simulink model "MBSE_system"  (R2022b)
settings: Solver=FixedStepDiscrete  StartTime=0.0  StopTime=10.0  RelTol=1e-3
settings Model: Creator=curro  LastModifiedBy=curro

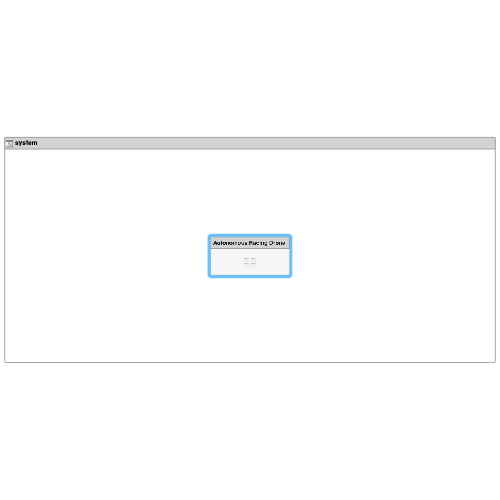
[thumbnail: Simulink's stored preview of the top-level diagram]
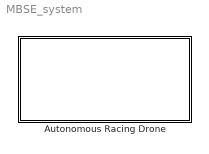
== system MBSE_system ==
  Autonomous Racing Drone : Subsystem
      settings: PortSchema="{\"entries\":[{\"content\":{\"headerSize\":26,\"margin\":15,\"minimumSpacing\":25,\"sides\":[{\"content\":{\"connectorIds\":[]},\"type\":\"ConnectorPlacement.EquallySpacedRectSide\",\"uuid\":\"710bb091-7129-4ee7-a780-76ad6f160d90\"},{\"content\":{\"connectorIds\":[],\"side\":\"RIGHT\"},\"type\":\"ConnectorPlacement.EquallySpacedRectSide\",\"uuid\":\"a14cb0ec-5ed5-4fd8-9e8a-b2c1d3079cde\"},{\"content\":{\"connectorIds\":[],\"side\":\"TOP\"},\"type\":\"ConnectorPlacement.EquallySpacedRectSide\",\"uuid\":\"b6825dff-2cae-452e-9344-6fbe12db9612\"}]},\"type\":\"ConnectorPlacement.EquallySpacedConnector\",\"uuid\":\"6fabdfc3-bcd5-4976-8a44-a7a5a39dd61e\"}],\"packageUris\":[\"http://schema.mathworks.com/mf0/Connector/R2020b\"],\"version\":\"1.0\"}"

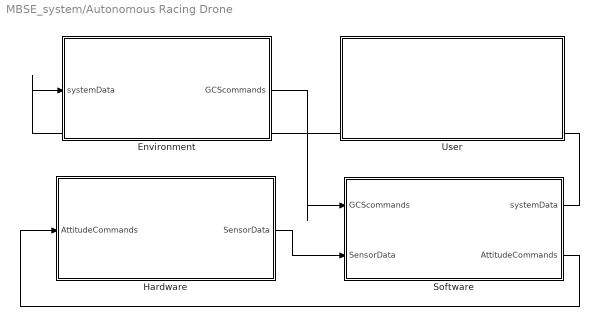
== system MBSE_system/Autonomous Racing Drone ==
  Environment : Subsystem
      settings: PortSchema="{\"entries\":[{\"content\":{\"headerSize\":26,\"margin\":15,\"minimumSpacing\":25,\"sides\":[{\"content\":{\"connectorIds\":[\"In1\"]},\"type\":\"ConnectorPlacement.EquallySpacedRectSide\",\"uuid\":\"710bb091-7129-4ee7-a780-76ad6f160d90\"},{\"content\":{\"connectorIds\":[\"Out1\"],\"side\":\"RIGHT\"},\"type\":\"ConnectorPlacement.EquallySpacedRectSide\",\"uuid\":\"a14cb0ec-5ed5-4fd8-9e8a-b2c1d3079cde\"},{\"content\":{\"connectorIds\":[],\"side\":\"TOP\"},\"type\":\"ConnectorPlacement.EquallySpacedRectSide\",\"uuid\":\"b6825dff-2cae-452e-9344-6fbe12db9612\"}]},\"type\":\"ConnectorPlacement.EquallySpacedConnector\",\"uuid\":\"6fabdfc3-bcd5-4976-8a44-a7a5a39dd61e\"}],\"packageUris\":[\"http://schema.mathworks.com/mf0/Connector/R2020b\"],\"version\":\"1.0\"}"
  Hardware : Subsystem
      settings: PortSchema="{\"entries\":[{\"content\":{\"headerSize\":26,\"margin\":15,\"minimumSpacing\":25,\"sides\":[{\"content\":{\"connectorIds\":[\"In1\"]},\"type\":\"ConnectorPlacement.EquallySpacedRectSide\",\"uuid\":\"710bb091-7129-4ee7-a780-76ad6f160d90\"},{\"content\":{\"connectorIds\":[\"Out1\"],\"side\":\"RIGHT\"},\"type\":\"ConnectorPlacement.EquallySpacedRectSide\",\"uuid\":\"a14cb0ec-5ed5-4fd8-9e8a-b2c1d3079cde\"},{\"content\":{\"connectorIds\":[],\"side\":\"TOP\"},\"type\":\"ConnectorPlacement.EquallySpacedRectSide\",\"uuid\":\"b6825dff-2cae-452e-9344-6fbe12db9612\"}]},\"type\":\"ConnectorPlacement.EquallySpacedConnector\",\"uuid\":\"6fabdfc3-bcd5-4976-8a44-a7a5a39dd61e\"}],\"packageUris\":[\"http://schema.mathworks.com/mf0/Connector/R2020b\"],\"version\":\"1.0\"}"
  Software : Subsystem
      settings: PortSchema="{\"entries\":[{\"content\":{\"headerSize\":26,\"margin\":15,\"minimumSpacing\":25,\"sides\":[{\"content\":{\"connectorIds\":[\"In2\",\"In1\"]},\"type\":\"ConnectorPlacement.EquallySpacedRectSide\",\"uuid\":\"710bb091-7129-4ee7-a780-76ad6f160d90\"},{\"content\":{\"connectorIds\":[\"Out1\",\"Out2\"],\"side\":\"RIGHT\"},\"type\":\"ConnectorPlacement.EquallySpacedRectSide\",\"uuid\":\"a14cb0ec-5ed5-4fd8-9e8a-b2c1d3079cde\"},{\"content\":{\"connectorIds\":[],\"side\":\"TOP\"},\"type\":\"ConnectorPlacement.EquallySpacedRectSide\",\"uuid\":\"b6825dff-2cae-452e-9344-6fbe12db9612\"}]},\"type\":\"ConnectorPlacement.EquallySpacedConnector\",\"uuid\":\"6fabdfc3-bcd5-4976-8a44-a7a5a39dd61e\"}],\"packageUris\":[\"http://schema.mathworks.com/mf0/Connector/R2020b\"],\"version\":\"1.0\"}"
  User : Subsystem
      settings: PortSchema="{\"entries\":[{\"content\":{\"headerSize\":26,\"margin\":15,\"minimumSpacing\":25,\"sides\":[{\"content\":{\"connectorIds\":[]},\"type\":\"ConnectorPlacement.EquallySpacedRectSide\",\"uuid\":\"710bb091-7129-4ee7-a780-76ad6f160d90\"},{\"content\":{\"connectorIds\":[],\"side\":\"RIGHT\"},\"type\":\"ConnectorPlacement.EquallySpacedRectSide\",\"uuid\":\"a14cb0ec-5ed5-4fd8-9e8a-b2c1d3079cde\"},{\"content\":{\"connectorIds\":[],\"side\":\"TOP\"},\"type\":\"ConnectorPlacement.EquallySpacedRectSide\",\"uuid\":\"b6825dff-2cae-452e-9344-6fbe12db9612\"}]},\"type\":\"ConnectorPlacement.EquallySpacedConnector\",\"uuid\":\"6fabdfc3-bcd5-4976-8a44-a7a5a39dd61e\"}],\"packageUris\":[\"http://schema.mathworks.com/mf0/Connector/R2020b\"],\"version\":\"1.0\"}"
  wires:
  Hardware/1(SensorData) -> Software/1(SensorData)
  Software/2(AttitudeCommands) -> Hardware/1(AttitudeCommands)
  Environment/1(GCScommands) -> Software/2(GCScommands)
  Software/1(systemData) -> Environment/1(systemData)

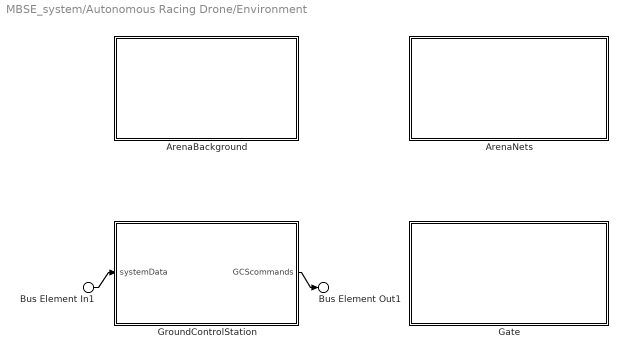
== system MBSE_system/Autonomous Racing Drone/Environment ==
  Bus Element In1 : Inport  PortName=systemData
  ArenaBackground : Subsystem
      settings: PortSchema="{\"entries\":[{\"content\":{\"headerSize\":26,\"margin\":15,\"minimumSpacing\":25,\"sides\":[{\"content\":{\"connectorIds\":[]},\"type\":\"ConnectorPlacement.EquallySpacedRectSide\",\"uuid\":\"710bb091-7129-4ee7-a780-76ad6f160d90\"},{\"content\":{\"connectorIds\":[],\"side\":\"RIGHT\"},\"type\":\"ConnectorPlacement.EquallySpacedRectSide\",\"uuid\":\"a14cb0ec-5ed5-4fd8-9e8a-b2c1d3079cde\"},{\"content\":{\"connectorIds\":[],\"side\":\"TOP\"},\"type\":\"ConnectorPlacement.EquallySpacedRectSide\",\"uuid\":\"b6825dff-2cae-452e-9344-6fbe12db9612\"}]},\"type\":\"ConnectorPlacement.EquallySpacedConnector\",\"uuid\":\"6fabdfc3-bcd5-4976-8a44-a7a5a39dd61e\"}],\"packageUris\":[\"http://schema.mathworks.com/mf0/Connector/R2020b\"],\"version\":\"1.0\"}"
  ArenaNets : Subsystem
      settings: PortSchema="{\"entries\":[{\"content\":{\"headerSize\":26,\"margin\":15,\"minimumSpacing\":25,\"sides\":[{\"content\":{\"connectorIds\":[]},\"type\":\"ConnectorPlacement.EquallySpacedRectSide\",\"uuid\":\"710bb091-7129-4ee7-a780-76ad6f160d90\"},{\"content\":{\"connectorIds\":[],\"side\":\"RIGHT\"},\"type\":\"ConnectorPlacement.EquallySpacedRectSide\",\"uuid\":\"a14cb0ec-5ed5-4fd8-9e8a-b2c1d3079cde\"},{\"content\":{\"connectorIds\":[],\"side\":\"TOP\"},\"type\":\"ConnectorPlacement.EquallySpacedRectSide\",\"uuid\":\"b6825dff-2cae-452e-9344-6fbe12db9612\"}]},\"type\":\"ConnectorPlacement.EquallySpacedConnector\",\"uuid\":\"6fabdfc3-bcd5-4976-8a44-a7a5a39dd61e\"}],\"packageUris\":[\"http://schema.mathworks.com/mf0/Connector/R2020b\"],\"version\":\"1.0\"}"
  Gate : Subsystem
      settings: PortSchema="{\"entries\":[{\"content\":{\"headerSize\":26,\"margin\":15,\"minimumSpacing\":25,\"sides\":[{\"content\":{\"connectorIds\":[]},\"type\":\"ConnectorPlacement.EquallySpacedRectSide\",\"uuid\":\"710bb091-7129-4ee7-a780-76ad6f160d90\"},{\"content\":{\"connectorIds\":[],\"side\":\"RIGHT\"},\"type\":\"ConnectorPlacement.EquallySpacedRectSide\",\"uuid\":\"a14cb0ec-5ed5-4fd8-9e8a-b2c1d3079cde\"},{\"content\":{\"connectorIds\":[],\"side\":\"TOP\"},\"type\":\"ConnectorPlacement.EquallySpacedRectSide\",\"uuid\":\"b6825dff-2cae-452e-9344-6fbe12db9612\"}]},\"type\":\"ConnectorPlacement.EquallySpacedConnector\",\"uuid\":\"6fabdfc3-bcd5-4976-8a44-a7a5a39dd61e\"}],\"packageUris\":[\"http://schema.mathworks.com/mf0/Connector/R2020b\"],\"version\":\"1.0\"}"
  GroundControlStation : Subsystem
      settings: PortSchema="{\"entries\":[{\"content\":{\"headerSize\":26,\"margin\":15,\"minimumSpacing\":25,\"sides\":[{\"content\":{\"connectorIds\":[\"In1\"]},\"type\":\"ConnectorPlacement.EquallySpacedRectSide\",\"uuid\":\"710bb091-7129-4ee7-a780-76ad6f160d90\"},{\"content\":{\"connectorIds\":[\"Out1\"],\"side\":\"RIGHT\"},\"type\":\"ConnectorPlacement.EquallySpacedRectSide\",\"uuid\":\"a14cb0ec-5ed5-4fd8-9e8a-b2c1d3079cde\"},{\"content\":{\"connectorIds\":[],\"side\":\"TOP\"},\"type\":\"ConnectorPlacement.EquallySpacedRectSide\",\"uuid\":\"b6825dff-2cae-452e-9344-6fbe12db9612\"}]},\"type\":\"ConnectorPlacement.EquallySpacedConnector\",\"uuid\":\"6fabdfc3-bcd5-4976-8a44-a7a5a39dd61e\"}],\"packageUris\":[\"http://schema.mathworks.com/mf0/Connector/R2020b\"],\"version\":\"1.0\"}"
  Bus Element Out1 : Outport  PortName=GCScommands
  wires:
  GroundControlStation/1(GCScommands) -> Bus Element Out1/1
  Bus Element In1/1 -> GroundControlStation/1(systemData)

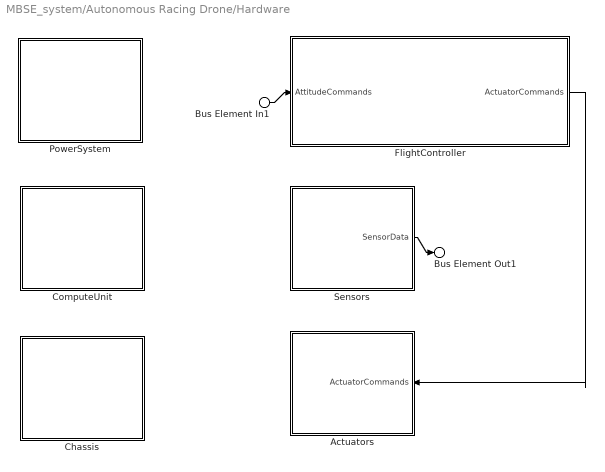
== system MBSE_system/Autonomous Racing Drone/Hardware ==
  Bus Element In1 : Inport  PortName=AttitudeCommands
  Actuators : Subsystem
      settings: PortSchema="{\"entries\":[{\"content\":{\"headerSize\":26,\"margin\":15,\"minimumSpacing\":25,\"sides\":[{\"content\":{\"connectorIds\":[]},\"type\":\"ConnectorPlacement.EquallySpacedRectSide\",\"uuid\":\"710bb091-7129-4ee7-a780-76ad6f160d90\"},{\"content\":{\"connectorIds\":[\"In1\"],\"side\":\"RIGHT\"},\"type\":\"ConnectorPlacement.EquallySpacedRectSide\",\"uuid\":\"a14cb0ec-5ed5-4fd8-9e8a-b2c1d3079cde\"},{\"content\":{\"connectorIds\":[],\"side\":\"TOP\"},\"type\":\"ConnectorPlacement.EquallySpacedRectSide\",\"uuid\":\"b6825dff-2cae-452e-9344-6fbe12db9612\"}]},\"type\":\"ConnectorPlacement.EquallySpacedConnector\",\"uuid\":\"6fabdfc3-bcd5-4976-8a44-a7a5a39dd61e\"}],\"packageUris\":[\"http://schema.mathworks.com/mf0/Connector/R2020b\"],\"version\":\"1.0\"}"
  Chassis : Subsystem
      settings: PortSchema="{\"entries\":[{\"content\":{\"headerSize\":26,\"margin\":15,\"minimumSpacing\":25,\"sides\":[{\"content\":{\"connectorIds\":[]},\"type\":\"ConnectorPlacement.EquallySpacedRectSide\",\"uuid\":\"710bb091-7129-4ee7-a780-76ad6f160d90\"},{\"content\":{\"connectorIds\":[],\"side\":\"RIGHT\"},\"type\":\"ConnectorPlacement.EquallySpacedRectSide\",\"uuid\":\"a14cb0ec-5ed5-4fd8-9e8a-b2c1d3079cde\"},{\"content\":{\"connectorIds\":[],\"side\":\"TOP\"},\"type\":\"ConnectorPlacement.EquallySpacedRectSide\",\"uuid\":\"b6825dff-2cae-452e-9344-6fbe12db9612\"}]},\"type\":\"ConnectorPlacement.EquallySpacedConnector\",\"uuid\":\"6fabdfc3-bcd5-4976-8a44-a7a5a39dd61e\"}],\"packageUris\":[\"http://schema.mathworks.com/mf0/Connector/R2020b\"],\"version\":\"1.0\"}"
  ComputeUnit : Subsystem
      settings: PortSchema="{\"entries\":[{\"content\":{\"headerSize\":26,\"margin\":15,\"minimumSpacing\":25,\"sides\":[{\"content\":{\"connectorIds\":[]},\"type\":\"ConnectorPlacement.EquallySpacedRectSide\",\"uuid\":\"710bb091-7129-4ee7-a780-76ad6f160d90\"},{\"content\":{\"connectorIds\":[],\"side\":\"RIGHT\"},\"type\":\"ConnectorPlacement.EquallySpacedRectSide\",\"uuid\":\"a14cb0ec-5ed5-4fd8-9e8a-b2c1d3079cde\"},{\"content\":{\"connectorIds\":[],\"side\":\"TOP\"},\"type\":\"ConnectorPlacement.EquallySpacedRectSide\",\"uuid\":\"b6825dff-2cae-452e-9344-6fbe12db9612\"}]},\"type\":\"ConnectorPlacement.EquallySpacedConnector\",\"uuid\":\"6fabdfc3-bcd5-4976-8a44-a7a5a39dd61e\"}],\"packageUris\":[\"http://schema.mathworks.com/mf0/Connector/R2020b\"],\"version\":\"1.0\"}"
  FlightController : Subsystem
      settings: PortSchema="{\"entries\":[{\"content\":{\"headerSize\":26,\"margin\":15,\"minimumSpacing\":25,\"sides\":[{\"content\":{\"connectorIds\":[\"In1\"]},\"type\":\"ConnectorPlacement.EquallySpacedRectSide\",\"uuid\":\"710bb091-7129-4ee7-a780-76ad6f160d90\"},{\"content\":{\"connectorIds\":[\"Out1\"],\"side\":\"RIGHT\"},\"type\":\"ConnectorPlacement.EquallySpacedRectSide\",\"uuid\":\"a14cb0ec-5ed5-4fd8-9e8a-b2c1d3079cde\"},{\"content\":{\"connectorIds\":[],\"side\":\"TOP\"},\"type\":\"ConnectorPlacement.EquallySpacedRectSide\",\"uuid\":\"b6825dff-2cae-452e-9344-6fbe12db9612\"}]},\"type\":\"ConnectorPlacement.EquallySpacedConnector\",\"uuid\":\"6fabdfc3-bcd5-4976-8a44-a7a5a39dd61e\"}],\"packageUris\":[\"http://schema.mathworks.com/mf0/Connector/R2020b\"],\"version\":\"1.0\"}"
  PowerSystem : Subsystem
      settings: PortSchema="{\"entries\":[{\"content\":{\"headerSize\":26,\"margin\":15,\"minimumSpacing\":25,\"sides\":[{\"content\":{\"connectorIds\":[]},\"type\":\"ConnectorPlacement.EquallySpacedRectSide\",\"uuid\":\"710bb091-7129-4ee7-a780-76ad6f160d90\"},{\"content\":{\"connectorIds\":[],\"side\":\"RIGHT\"},\"type\":\"ConnectorPlacement.EquallySpacedRectSide\",\"uuid\":\"a14cb0ec-5ed5-4fd8-9e8a-b2c1d3079cde\"},{\"content\":{\"connectorIds\":[],\"side\":\"TOP\"},\"type\":\"ConnectorPlacement.EquallySpacedRectSide\",\"uuid\":\"b6825dff-2cae-452e-9344-6fbe12db9612\"}]},\"type\":\"ConnectorPlacement.EquallySpacedConnector\",\"uuid\":\"6fabdfc3-bcd5-4976-8a44-a7a5a39dd61e\"}],\"packageUris\":[\"http://schema.mathworks.com/mf0/Connector/R2020b\"],\"version\":\"1.0\"}"
  Sensors : Subsystem
      settings: PortSchema="{\"entries\":[{\"content\":{\"headerSize\":26,\"margin\":15,\"minimumSpacing\":25,\"sides\":[{\"content\":{\"connectorIds\":[]},\"type\":\"ConnectorPlacement.EquallySpacedRectSide\",\"uuid\":\"710bb091-7129-4ee7-a780-76ad6f160d90\"},{\"content\":{\"connectorIds\":[\"Out1\"],\"side\":\"RIGHT\"},\"type\":\"ConnectorPlacement.EquallySpacedRectSide\",\"uuid\":\"a14cb0ec-5ed5-4fd8-9e8a-b2c1d3079cde\"},{\"content\":{\"connectorIds\":[],\"side\":\"TOP\"},\"type\":\"ConnectorPlacement.EquallySpacedRectSide\",\"uuid\":\"b6825dff-2cae-452e-9344-6fbe12db9612\"}]},\"type\":\"ConnectorPlacement.EquallySpacedConnector\",\"uuid\":\"6fabdfc3-bcd5-4976-8a44-a7a5a39dd61e\"}],\"packageUris\":[\"http://schema.mathworks.com/mf0/Connector/R2020b\"],\"version\":\"1.0\"}"
  Bus Element Out1 : Outport  PortName=SensorData
  wires:
  Sensors/1(SensorData) -> Bus Element Out1/1
  FlightController/1(ActuatorCommands) -> Actuators/1(ActuatorCommands)
  Bus Element In1/1 -> FlightController/1(AttitudeCommands)

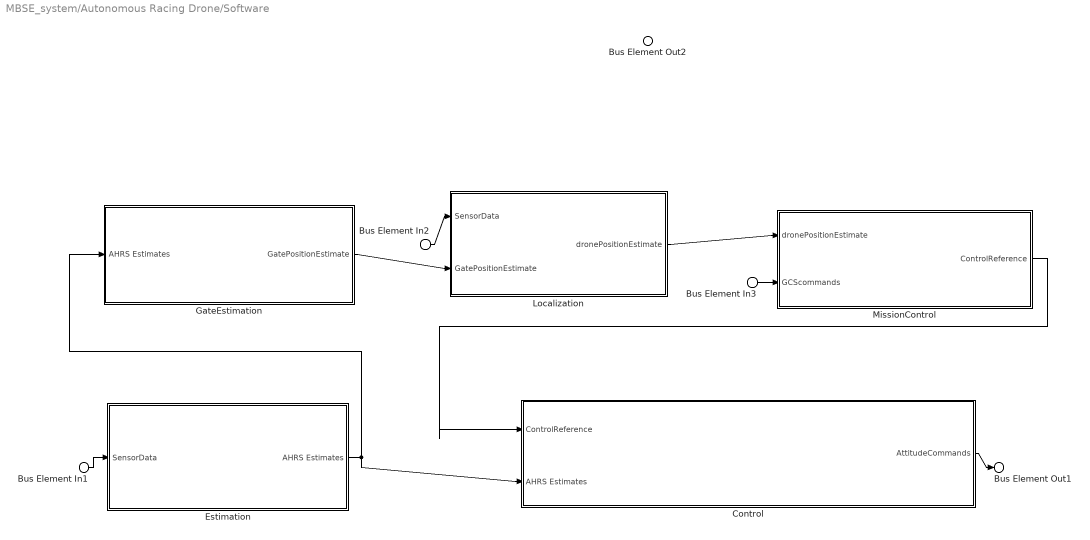
== system MBSE_system/Autonomous Racing Drone/Software ==
  Bus Element In1 : Inport  PortName=SensorData
  Bus Element In2 : Inport  PortName=SensorData
  Bus Element In3 : Inport  Port=2  PortName=GCScommands
  Control : Subsystem
      settings: PortSchema="{\"entries\":[{\"content\":{\"headerSize\":26,\"margin\":15,\"minimumSpacing\":25,\"sides\":[{\"content\":{\"connectorIds\":[\"In2\",\"In1\"]},\"type\":\"ConnectorPlacement.EquallySpacedRectSide\",\"uuid\":\"710bb091-7129-4ee7-a780-76ad6f160d90\"},{\"content\":{\"connectorIds\":[\"Out1\"],\"side\":\"RIGHT\"},\"type\":\"ConnectorPlacement.EquallySpacedRectSide\",\"uuid\":\"a14cb0ec-5ed5-4fd8-9e8a-b2c1d3079cde\"},{\"content\":{\"connectorIds\":[],\"side\":\"TOP\"},\"type\":\"ConnectorPlacement.EquallySpacedRectSide\",\"uuid\":\"b6825dff-2cae-452e-9344-6fbe12db9612\"}]},\"type\":\"ConnectorPlacement.EquallySpacedConnector\",\"uuid\":\"6fabdfc3-bcd5-4976-8a44-a7a5a39dd61e\"}],\"packageUris\":[\"http://schema.mathworks.com/mf0/Connector/R2020b\"],\"version\":\"1.0\"}"
  Estimation : Subsystem
      settings: PortSchema="{\"entries\":[{\"content\":{\"headerSize\":26,\"margin\":15,\"minimumSpacing\":25,\"sides\":[{\"content\":{\"connectorIds\":[\"In1\"]},\"type\":\"ConnectorPlacement.EquallySpacedRectSide\",\"uuid\":\"710bb091-7129-4ee7-a780-76ad6f160d90\"},{\"content\":{\"connectorIds\":[\"Out1\"],\"side\":\"RIGHT\"},\"type\":\"ConnectorPlacement.EquallySpacedRectSide\",\"uuid\":\"a14cb0ec-5ed5-4fd8-9e8a-b2c1d3079cde\"},{\"content\":{\"connectorIds\":[],\"side\":\"TOP\"},\"type\":\"ConnectorPlacement.EquallySpacedRectSide\",\"uuid\":\"b6825dff-2cae-452e-9344-6fbe12db9612\"},{\"content\":{\"connectorIds\":[],\"side\":\"BOTTOM\"},\"type\":\"ConnectorPlacement.EquallySpacedRectSide\",\"uuid\":\"9d5a03c7-b76b-46f7-929d-e8cb0e1dbaac\"}]},\"type\":\"ConnectorPlacement.EquallySpacedConnector\",\"uuid\":\"6fabdfc3-bcd5-4976-8a44-a7a5a39dd61e\"}],\"packageUris\":[\"http://schema.mathworks.com/mf0/Connector/R2020b\"],\"version\":\"1.0\"}"
  GateEstimation : Subsystem
      settings: PortSchema="{\"entries\":[{\"content\":{\"headerSize\":26,\"margin\":15,\"minimumSpacing\":25,\"sides\":[{\"content\":{\"connectorIds\":[\"In1\"]},\"type\":\"ConnectorPlacement.EquallySpacedRectSide\",\"uuid\":\"710bb091-7129-4ee7-a780-76ad6f160d90\"},{\"content\":{\"connectorIds\":[\"Out1\"],\"side\":\"RIGHT\"},\"type\":\"ConnectorPlacement.EquallySpacedRectSide\",\"uuid\":\"a14cb0ec-5ed5-4fd8-9e8a-b2c1d3079cde\"},{\"content\":{\"connectorIds\":[],\"side\":\"TOP\"},\"type\":\"ConnectorPlacement.EquallySpacedRectSide\",\"uuid\":\"b6825dff-2cae-452e-9344-6fbe12db9612\"}]},\"type\":\"ConnectorPlacement.EquallySpacedConnector\",\"uuid\":\"6fabdfc3-bcd5-4976-8a44-a7a5a39dd61e\"}],\"packageUris\":[\"http://schema.mathworks.com/mf0/Connector/R2020b\"],\"version\":\"1.0\"}"
  Localization : Subsystem
      settings: PortSchema="{\"entries\":[{\"content\":{\"headerSize\":26,\"margin\":15,\"minimumSpacing\":25,\"sides\":[{\"content\":{\"connectorIds\":[\"In1\",\"In2\"]},\"type\":\"ConnectorPlacement.EquallySpacedRectSide\",\"uuid\":\"710bb091-7129-4ee7-a780-76ad6f160d90\"},{\"content\":{\"connectorIds\":[\"Out1\"],\"side\":\"RIGHT\"},\"type\":\"ConnectorPlacement.EquallySpacedRectSide\",\"uuid\":\"a14cb0ec-5ed5-4fd8-9e8a-b2c1d3079cde\"},{\"content\":{\"connectorIds\":[],\"side\":\"TOP\"},\"type\":\"ConnectorPlacement.EquallySpacedRectSide\",\"uuid\":\"b6825dff-2cae-452e-9344-6fbe12db9612\"}]},\"type\":\"ConnectorPlacement.EquallySpacedConnector\",\"uuid\":\"6fabdfc3-bcd5-4976-8a44-a7a5a39dd61e\"}],\"packageUris\":[\"http://schema.mathworks.com/mf0/Connector/R2020b\"],\"version\":\"1.0\"}"
  MissionControl : Subsystem
      settings: PortSchema="{\"entries\":[{\"content\":{\"headerSize\":26,\"margin\":15,\"minimumSpacing\":25,\"sides\":[{\"content\":{\"connectorIds\":[\"In1\",\"In2\"]},\"type\":\"ConnectorPlacement.EquallySpacedRectSide\",\"uuid\":\"710bb091-7129-4ee7-a780-76ad6f160d90\"},{\"content\":{\"connectorIds\":[\"Out1\"],\"side\":\"RIGHT\"},\"type\":\"ConnectorPlacement.EquallySpacedRectSide\",\"uuid\":\"a14cb0ec-5ed5-4fd8-9e8a-b2c1d3079cde\"},{\"content\":{\"connectorIds\":[],\"side\":\"TOP\"},\"type\":\"ConnectorPlacement.EquallySpacedRectSide\",\"uuid\":\"b6825dff-2cae-452e-9344-6fbe12db9612\"}]},\"type\":\"ConnectorPlacement.EquallySpacedConnector\",\"uuid\":\"6fabdfc3-bcd5-4976-8a44-a7a5a39dd61e\"}],\"packageUris\":[\"http://schema.mathworks.com/mf0/Connector/R2020b\"],\"version\":\"1.0\"}"
  Bus Element Out2 : Outport  PortName=systemData
  Bus Element Out1 : Outport  Port=2  PortName=AttitudeCommands
  wires:
  Bus Element In1/1 -> Estimation/1(SensorData)
  GateEstimation/1(GatePositionEstimate) -> Localization/2(GatePositionEstimate)
  MissionControl/1(ControlReference) -> Control/2(ControlReference)
  Estimation/1(AHRS Estimates) -> Control/1(AHRS Estimates), GateEstimation/1(AHRS Estimates)
  Bus Element In2/1 -> Localization/1(SensorData)
  Control/1(AttitudeCommands) -> Bus Element Out1/1
  Bus Element In3/1 -> MissionControl/2(GCScommands)
  Localization/1(dronePositionEstimate) -> MissionControl/1(dronePositionEstimate)

== system MBSE_system/Autonomous Racing Drone/User ==
  Team operators : Subsystem
      settings: PortSchema="{\"entries\":[{\"content\":{\"headerSize\":26,\"margin\":15,\"minimumSpacing\":25,\"sides\":[{\"content\":{\"connectorIds\":[]},\"type\":\"ConnectorPlacement.EquallySpacedRectSide\",\"uuid\":\"710bb091-7129-4ee7-a780-76ad6f160d90\"},{\"content\":{\"connectorIds\":[],\"side\":\"RIGHT\"},\"type\":\"ConnectorPlacement.EquallySpacedRectSide\",\"uuid\":\"a14cb0ec-5ed5-4fd8-9e8a-b2c1d3079cde\"},{\"content\":{\"connectorIds\":[],\"side\":\"TOP\"},\"type\":\"ConnectorPlacement.EquallySpacedRectSide\",\"uuid\":\"b6825dff-2cae-452e-9344-6fbe12db9612\"}]},\"type\":\"ConnectorPlacement.EquallySpacedConnector\",\"uuid\":\"6fabdfc3-bcd5-4976-8a44-a7a5a39dd61e\"}],\"packageUris\":[\"http://schema.mathworks.com/mf0/Connector/R2020b\"],\"version\":\"1.0\"}"

== system MBSE_system/Autonomous Racing Drone/Environment/ArenaBackground ==

== system MBSE_system/Autonomous Racing Drone/Environment/ArenaNets ==

== system MBSE_system/Autonomous Racing Drone/Environment/Gate ==

== system MBSE_system/Autonomous Racing Drone/Environment/GroundControlStation ==
  Bus Element In1 : Inport  PortName=systemData
  Bus Element Out1 : Outport  PortName=GCScommands

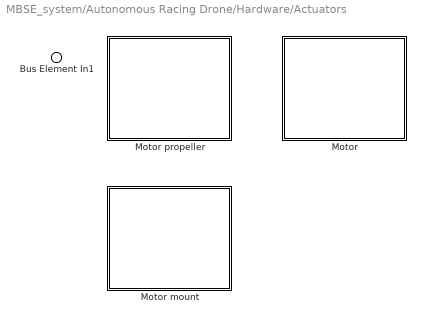
== system MBSE_system/Autonomous Racing Drone/Hardware/Actuators ==
  Bus Element In1 : Inport  PortName=ActuatorCommands
  Motor : Subsystem
      settings: PortSchema="{\"entries\":[{\"content\":{\"headerSize\":26,\"margin\":15,\"minimumSpacing\":25,\"sides\":[{\"content\":{\"connectorIds\":[]},\"type\":\"ConnectorPlacement.EquallySpacedRectSide\",\"uuid\":\"710bb091-7129-4ee7-a780-76ad6f160d90\"},{\"content\":{\"connectorIds\":[],\"side\":\"RIGHT\"},\"type\":\"ConnectorPlacement.EquallySpacedRectSide\",\"uuid\":\"a14cb0ec-5ed5-4fd8-9e8a-b2c1d3079cde\"},{\"content\":{\"connectorIds\":[],\"side\":\"TOP\"},\"type\":\"ConnectorPlacement.EquallySpacedRectSide\",\"uuid\":\"b6825dff-2cae-452e-9344-6fbe12db9612\"}]},\"type\":\"ConnectorPlacement.EquallySpacedConnector\",\"uuid\":\"6fabdfc3-bcd5-4976-8a44-a7a5a39dd61e\"}],\"packageUris\":[\"http://schema.mathworks.com/mf0/Connector/R2020b\"],\"version\":\"1.0\"}"
  Motor mount : Subsystem
      settings: PortSchema="{\"entries\":[{\"content\":{\"headerSize\":26,\"margin\":15,\"minimumSpacing\":25,\"sides\":[{\"content\":{\"connectorIds\":[]},\"type\":\"ConnectorPlacement.EquallySpacedRectSide\",\"uuid\":\"710bb091-7129-4ee7-a780-76ad6f160d90\"},{\"content\":{\"connectorIds\":[],\"side\":\"RIGHT\"},\"type\":\"ConnectorPlacement.EquallySpacedRectSide\",\"uuid\":\"a14cb0ec-5ed5-4fd8-9e8a-b2c1d3079cde\"},{\"content\":{\"connectorIds\":[],\"side\":\"TOP\"},\"type\":\"ConnectorPlacement.EquallySpacedRectSide\",\"uuid\":\"b6825dff-2cae-452e-9344-6fbe12db9612\"}]},\"type\":\"ConnectorPlacement.EquallySpacedConnector\",\"uuid\":\"6fabdfc3-bcd5-4976-8a44-a7a5a39dd61e\"}],\"packageUris\":[\"http://schema.mathworks.com/mf0/Connector/R2020b\"],\"version\":\"1.0\"}"
  Motor propeller : Subsystem
      settings: PortSchema="{\"entries\":[{\"content\":{\"headerSize\":26,\"margin\":15,\"minimumSpacing\":25,\"sides\":[{\"content\":{\"connectorIds\":[]},\"type\":\"ConnectorPlacement.EquallySpacedRectSide\",\"uuid\":\"710bb091-7129-4ee7-a780-76ad6f160d90\"},{\"content\":{\"connectorIds\":[],\"side\":\"RIGHT\"},\"type\":\"ConnectorPlacement.EquallySpacedRectSide\",\"uuid\":\"a14cb0ec-5ed5-4fd8-9e8a-b2c1d3079cde\"},{\"content\":{\"connectorIds\":[],\"side\":\"TOP\"},\"type\":\"ConnectorPlacement.EquallySpacedRectSide\",\"uuid\":\"b6825dff-2cae-452e-9344-6fbe12db9612\"}]},\"type\":\"ConnectorPlacement.EquallySpacedConnector\",\"uuid\":\"6fabdfc3-bcd5-4976-8a44-a7a5a39dd61e\"}],\"packageUris\":[\"http://schema.mathworks.com/mf0/Connector/R2020b\"],\"version\":\"1.0\"}"

== system MBSE_system/Autonomous Racing Drone/Hardware/Chassis ==

== system MBSE_system/Autonomous Racing Drone/Hardware/ComputeUnit ==

== system MBSE_system/Autonomous Racing Drone/Hardware/FlightController ==
  Bus Element In1 : Inport  PortName=AttitudeCommands
  Bus Element Out1 : Outport  PortName=ActuatorCommands

== system MBSE_system/Autonomous Racing Drone/Hardware/PowerSystem ==

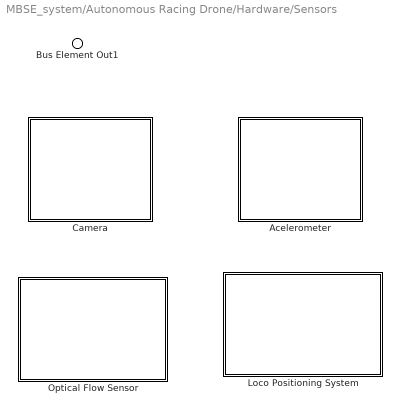
== system MBSE_system/Autonomous Racing Drone/Hardware/Sensors ==
  Acelerometer : Subsystem
      settings: PortSchema="{\"entries\":[{\"content\":{\"headerSize\":26,\"margin\":15,\"minimumSpacing\":25,\"sides\":[{\"content\":{\"connectorIds\":[]},\"type\":\"ConnectorPlacement.EquallySpacedRectSide\",\"uuid\":\"710bb091-7129-4ee7-a780-76ad6f160d90\"},{\"content\":{\"connectorIds\":[],\"side\":\"RIGHT\"},\"type\":\"ConnectorPlacement.EquallySpacedRectSide\",\"uuid\":\"a14cb0ec-5ed5-4fd8-9e8a-b2c1d3079cde\"},{\"content\":{\"connectorIds\":[],\"side\":\"TOP\"},\"type\":\"ConnectorPlacement.EquallySpacedRectSide\",\"uuid\":\"b6825dff-2cae-452e-9344-6fbe12db9612\"}]},\"type\":\"ConnectorPlacement.EquallySpacedConnector\",\"uuid\":\"6fabdfc3-bcd5-4976-8a44-a7a5a39dd61e\"}],\"packageUris\":[\"http://schema.mathworks.com/mf0/Connector/R2020b\"],\"version\":\"1.0\"}"
  Camera : Subsystem
      settings: PortSchema="{\"entries\":[{\"content\":{\"headerSize\":26,\"margin\":15,\"minimumSpacing\":25,\"sides\":[{\"content\":{\"connectorIds\":[]},\"type\":\"ConnectorPlacement.EquallySpacedRectSide\",\"uuid\":\"710bb091-7129-4ee7-a780-76ad6f160d90\"},{\"content\":{\"connectorIds\":[],\"side\":\"RIGHT\"},\"type\":\"ConnectorPlacement.EquallySpacedRectSide\",\"uuid\":\"a14cb0ec-5ed5-4fd8-9e8a-b2c1d3079cde\"},{\"content\":{\"connectorIds\":[],\"side\":\"TOP\"},\"type\":\"ConnectorPlacement.EquallySpacedRectSide\",\"uuid\":\"b6825dff-2cae-452e-9344-6fbe12db9612\"}]},\"type\":\"ConnectorPlacement.EquallySpacedConnector\",\"uuid\":\"6fabdfc3-bcd5-4976-8a44-a7a5a39dd61e\"}],\"packageUris\":[\"http://schema.mathworks.com/mf0/Connector/R2020b\"],\"version\":\"1.0\"}"
  Loco Positioning System : Subsystem
      settings: PortSchema="{\"entries\":[{\"content\":{\"headerSize\":26,\"margin\":15,\"minimumSpacing\":25,\"sides\":[{\"content\":{\"connectorIds\":[]},\"type\":\"ConnectorPlacement.EquallySpacedRectSide\",\"uuid\":\"710bb091-7129-4ee7-a780-76ad6f160d90\"},{\"content\":{\"connectorIds\":[],\"side\":\"RIGHT\"},\"type\":\"ConnectorPlacement.EquallySpacedRectSide\",\"uuid\":\"a14cb0ec-5ed5-4fd8-9e8a-b2c1d3079cde\"},{\"content\":{\"connectorIds\":[],\"side\":\"TOP\"},\"type\":\"ConnectorPlacement.EquallySpacedRectSide\",\"uuid\":\"b6825dff-2cae-452e-9344-6fbe12db9612\"}]},\"type\":\"ConnectorPlacement.EquallySpacedConnector\",\"uuid\":\"6fabdfc3-bcd5-4976-8a44-a7a5a39dd61e\"}],\"packageUris\":[\"http://schema.mathworks.com/mf0/Connector/R2020b\"],\"version\":\"1.0\"}"
  Optical Flow Sensor : Subsystem
      settings: PortSchema="{\"entries\":[{\"content\":{\"headerSize\":26,\"margin\":15,\"minimumSpacing\":25,\"sides\":[{\"content\":{\"connectorIds\":[]},\"type\":\"ConnectorPlacement.EquallySpacedRectSide\",\"uuid\":\"710bb091-7129-4ee7-a780-76ad6f160d90\"},{\"content\":{\"connectorIds\":[],\"side\":\"RIGHT\"},\"type\":\"ConnectorPlacement.EquallySpacedRectSide\",\"uuid\":\"a14cb0ec-5ed5-4fd8-9e8a-b2c1d3079cde\"},{\"content\":{\"connectorIds\":[],\"side\":\"TOP\"},\"type\":\"ConnectorPlacement.EquallySpacedRectSide\",\"uuid\":\"b6825dff-2cae-452e-9344-6fbe12db9612\"}]},\"type\":\"ConnectorPlacement.EquallySpacedConnector\",\"uuid\":\"6fabdfc3-bcd5-4976-8a44-a7a5a39dd61e\"}],\"packageUris\":[\"http://schema.mathworks.com/mf0/Connector/R2020b\"],\"version\":\"1.0\"}"
  Bus Element Out1 : Outport  PortName=SensorData

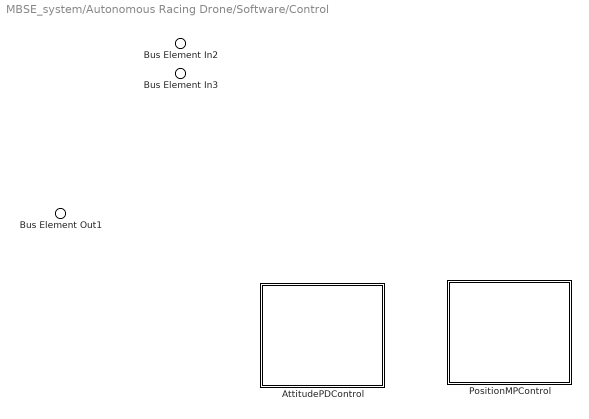
== system MBSE_system/Autonomous Racing Drone/Software/Control ==
  Bus Element In3 : Inport  PortName=AHRS Estimates
  Bus Element In2 : Inport  Port=2  PortName=ControlReference
  AttitudePDControl : Subsystem
      settings: PortSchema="{\"entries\":[{\"content\":{\"headerSize\":26,\"margin\":15,\"minimumSpacing\":25,\"sides\":[{\"content\":{\"connectorIds\":[]},\"type\":\"ConnectorPlacement.EquallySpacedRectSide\",\"uuid\":\"710bb091-7129-4ee7-a780-76ad6f160d90\"},{\"content\":{\"connectorIds\":[],\"side\":\"RIGHT\"},\"type\":\"ConnectorPlacement.EquallySpacedRectSide\",\"uuid\":\"a14cb0ec-5ed5-4fd8-9e8a-b2c1d3079cde\"},{\"content\":{\"connectorIds\":[],\"side\":\"TOP\"},\"type\":\"ConnectorPlacement.EquallySpacedRectSide\",\"uuid\":\"b6825dff-2cae-452e-9344-6fbe12db9612\"}]},\"type\":\"ConnectorPlacement.EquallySpacedConnector\",\"uuid\":\"6fabdfc3-bcd5-4976-8a44-a7a5a39dd61e\"}],\"packageUris\":[\"http://schema.mathworks.com/mf0/Connector/R2020b\"],\"version\":\"1.0\"}"
  PositionMPControl : Subsystem
      settings: PortSchema="{\"entries\":[{\"content\":{\"headerSize\":26,\"margin\":15,\"minimumSpacing\":25,\"sides\":[{\"content\":{\"connectorIds\":[]},\"type\":\"ConnectorPlacement.EquallySpacedRectSide\",\"uuid\":\"710bb091-7129-4ee7-a780-76ad6f160d90\"},{\"content\":{\"connectorIds\":[],\"side\":\"RIGHT\"},\"type\":\"ConnectorPlacement.EquallySpacedRectSide\",\"uuid\":\"a14cb0ec-5ed5-4fd8-9e8a-b2c1d3079cde\"},{\"content\":{\"connectorIds\":[],\"side\":\"TOP\"},\"type\":\"ConnectorPlacement.EquallySpacedRectSide\",\"uuid\":\"b6825dff-2cae-452e-9344-6fbe12db9612\"}]},\"type\":\"ConnectorPlacement.EquallySpacedConnector\",\"uuid\":\"6fabdfc3-bcd5-4976-8a44-a7a5a39dd61e\"}],\"packageUris\":[\"http://schema.mathworks.com/mf0/Connector/R2020b\"],\"version\":\"1.0\"}"
  Bus Element Out1 : Outport  PortName=AttitudeCommands

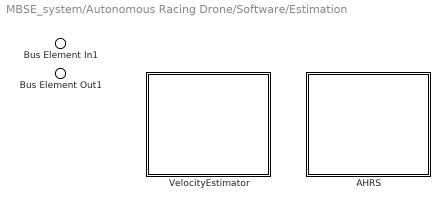
== system MBSE_system/Autonomous Racing Drone/Software/Estimation ==
  Bus Element In1 : Inport  PortName=SensorData
  AHRS : Subsystem
      settings: PortSchema="{\"entries\":[{\"content\":{\"headerSize\":26,\"margin\":15,\"minimumSpacing\":25,\"sides\":[{\"content\":{\"connectorIds\":[]},\"type\":\"ConnectorPlacement.EquallySpacedRectSide\",\"uuid\":\"710bb091-7129-4ee7-a780-76ad6f160d90\"},{\"content\":{\"connectorIds\":[],\"side\":\"RIGHT\"},\"type\":\"ConnectorPlacement.EquallySpacedRectSide\",\"uuid\":\"a14cb0ec-5ed5-4fd8-9e8a-b2c1d3079cde\"},{\"content\":{\"connectorIds\":[],\"side\":\"TOP\"},\"type\":\"ConnectorPlacement.EquallySpacedRectSide\",\"uuid\":\"b6825dff-2cae-452e-9344-6fbe12db9612\"}]},\"type\":\"ConnectorPlacement.EquallySpacedConnector\",\"uuid\":\"6fabdfc3-bcd5-4976-8a44-a7a5a39dd61e\"}],\"packageUris\":[\"http://schema.mathworks.com/mf0/Connector/R2020b\"],\"version\":\"1.0\"}"
  VelocityEstimator : Subsystem
      settings: PortSchema="{\"entries\":[{\"content\":{\"headerSize\":26,\"margin\":15,\"minimumSpacing\":25,\"sides\":[{\"content\":{\"connectorIds\":[]},\"type\":\"ConnectorPlacement.EquallySpacedRectSide\",\"uuid\":\"710bb091-7129-4ee7-a780-76ad6f160d90\"},{\"content\":{\"connectorIds\":[],\"side\":\"RIGHT\"},\"type\":\"ConnectorPlacement.EquallySpacedRectSide\",\"uuid\":\"a14cb0ec-5ed5-4fd8-9e8a-b2c1d3079cde\"},{\"content\":{\"connectorIds\":[],\"side\":\"TOP\"},\"type\":\"ConnectorPlacement.EquallySpacedRectSide\",\"uuid\":\"b6825dff-2cae-452e-9344-6fbe12db9612\"}]},\"type\":\"ConnectorPlacement.EquallySpacedConnector\",\"uuid\":\"6fabdfc3-bcd5-4976-8a44-a7a5a39dd61e\"}],\"packageUris\":[\"http://schema.mathworks.com/mf0/Connector/R2020b\"],\"version\":\"1.0\"}"
  Bus Element Out1 : Outport  PortName=AHRS Estimates

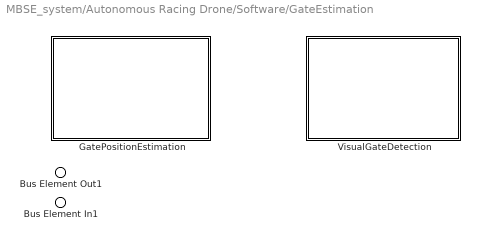
== system MBSE_system/Autonomous Racing Drone/Software/GateEstimation ==
  Bus Element In1 : Inport  PortName=AHRS Estimates
  GatePositionEstimation : Subsystem
      settings: PortSchema="{\"entries\":[{\"content\":{\"headerSize\":26,\"margin\":15,\"minimumSpacing\":25,\"sides\":[{\"content\":{\"connectorIds\":[]},\"type\":\"ConnectorPlacement.EquallySpacedRectSide\",\"uuid\":\"710bb091-7129-4ee7-a780-76ad6f160d90\"},{\"content\":{\"connectorIds\":[],\"side\":\"RIGHT\"},\"type\":\"ConnectorPlacement.EquallySpacedRectSide\",\"uuid\":\"a14cb0ec-5ed5-4fd8-9e8a-b2c1d3079cde\"},{\"content\":{\"connectorIds\":[],\"side\":\"TOP\"},\"type\":\"ConnectorPlacement.EquallySpacedRectSide\",\"uuid\":\"b6825dff-2cae-452e-9344-6fbe12db9612\"}]},\"type\":\"ConnectorPlacement.EquallySpacedConnector\",\"uuid\":\"6fabdfc3-bcd5-4976-8a44-a7a5a39dd61e\"}],\"packageUris\":[\"http://schema.mathworks.com/mf0/Connector/R2020b\"],\"version\":\"1.0\"}"
  VisualGateDetection : Subsystem
      settings: PortSchema="{\"entries\":[{\"content\":{\"headerSize\":26,\"margin\":15,\"minimumSpacing\":25,\"sides\":[{\"content\":{\"connectorIds\":[]},\"type\":\"ConnectorPlacement.EquallySpacedRectSide\",\"uuid\":\"710bb091-7129-4ee7-a780-76ad6f160d90\"},{\"content\":{\"connectorIds\":[],\"side\":\"RIGHT\"},\"type\":\"ConnectorPlacement.EquallySpacedRectSide\",\"uuid\":\"a14cb0ec-5ed5-4fd8-9e8a-b2c1d3079cde\"},{\"content\":{\"connectorIds\":[],\"side\":\"TOP\"},\"type\":\"ConnectorPlacement.EquallySpacedRectSide\",\"uuid\":\"b6825dff-2cae-452e-9344-6fbe12db9612\"}]},\"type\":\"ConnectorPlacement.EquallySpacedConnector\",\"uuid\":\"6fabdfc3-bcd5-4976-8a44-a7a5a39dd61e\"}],\"packageUris\":[\"http://schema.mathworks.com/mf0/Connector/R2020b\"],\"version\":\"1.0\"}"
  Bus Element Out1 : Outport  PortName=GatePositionEstimate

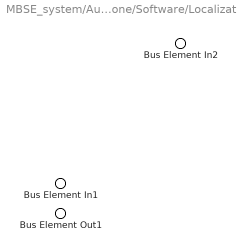
== system MBSE_system/Autonomous Racing Drone/Software/Localization ==
  Bus Element In2 : Inport  PortName=SensorData
  Bus Element In1 : Inport  Port=2  PortName=GatePositionEstimate
  Bus Element Out1 : Outport  PortName=dronePositionEstimate

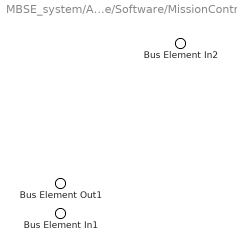
== system MBSE_system/Autonomous Racing Drone/Software/MissionControl ==
  Bus Element In2 : Inport  PortName=dronePositionEstimate
  Bus Element In1 : Inport  Port=2  PortName=GCScommands
  Bus Element Out1 : Outport  PortName=ControlReference

== system MBSE_system/Autonomous Racing Drone/User/Team operators ==

== system MBSE_system/Autonomous Racing Drone/Hardware/Actuators/Motor ==

== system MBSE_system/Autonomous Racing Drone/Hardware/Actuators/Motor mount ==

== system MBSE_system/Autonomous Racing Drone/Hardware/Actuators/Motor propeller ==

== system MBSE_system/Autonomous Racing Drone/Hardware/Sensors/Acelerometer ==

== system MBSE_system/Autonomous Racing Drone/Hardware/Sensors/Camera ==

== system MBSE_system/Autonomous Racing Drone/Hardware/Sensors/Loco Positioning System ==

== system MBSE_system/Autonomous Racing Drone/Hardware/Sensors/Optical Flow Sensor ==

== system MBSE_system/Autonomous Racing Drone/Software/Control/AttitudePDControl ==

== system MBSE_system/Autonomous Racing Drone/Software/Control/PositionMPControl ==

== system MBSE_system/Autonomous Racing Drone/Software/Estimation/AHRS ==

== system MBSE_system/Autonomous Racing Drone/Software/Estimation/VelocityEstimator ==

== system MBSE_system/Autonomous Racing Drone/Software/GateEstimation/GatePositionEstimation ==

== system MBSE_system/Autonomous Racing Drone/Software/GateEstimation/VisualGateDetection ==
